simulink model "sim_PD"  (R2023a)
settings: Solver=VariableStepAuto  StartTime=0.0  StopTime=20  RelTol=1e-3
values from neighbouring files (symbols this model uses):
  Kd = ((4*Jeff)/A-Beff)/Km_R    [val.m]
  Kp = (4*Jeff)/(square(A)*Km_R)    [val.m]
  r = 1/200    (= 0.005)    [val.m]
libraries: lib_robotRP_new x2
settings Model: Creator=gbl3344a  LastModifiedBy=gbl3344a

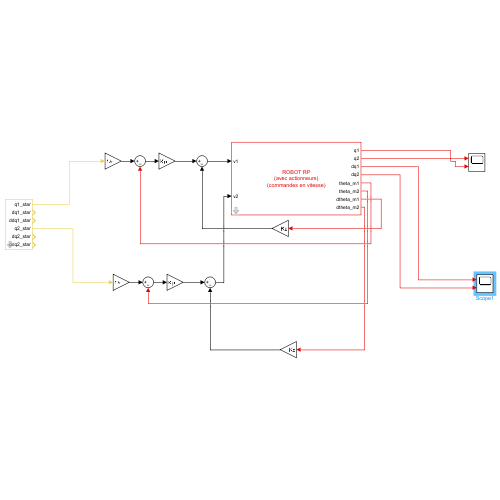
[thumbnail: Simulink's stored preview of the top-level diagram]
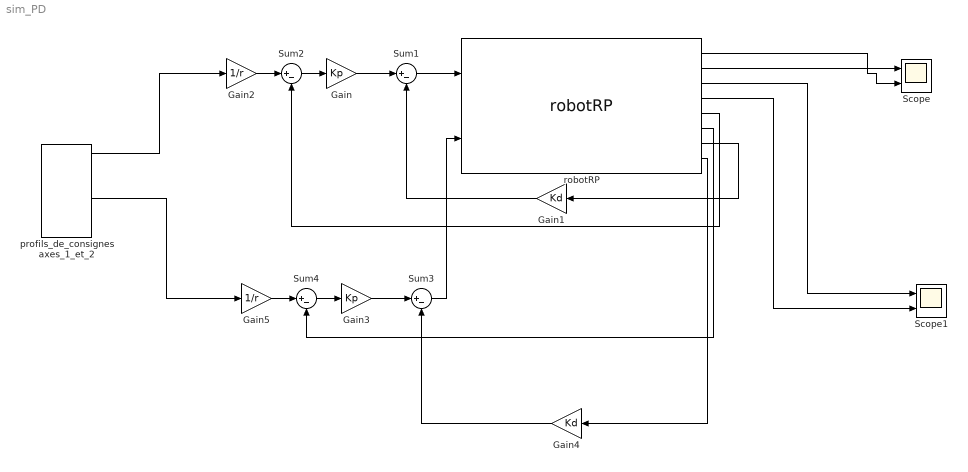
== system sim_PD ==
  Gain : Gain  Gain=Kp
  Gain1 : Gain  Gain=Kd
  Gain2 : Gain  Gain=1/r
  Gain3 : Gain  Gain=Kp
  Gain4 : Gain  Gain=Kd
  Gain5 : Gain  Gain=1/r
  Scope : Scope  NumInputPorts=2
  Scope1 : Scope  NumInputPorts=2
  Sum{1..4} (4 alike) : Sum  Inputs=|+-
  profils_de_consignes axes_1_et_2 : lib_robotRP_new/profils_de_consignes axes_1_et_2
  robotRP : lib_robotRP_new/robotRP  vecteur_theta_dtheta_initial=[0 ; 100 ; 0 ; 0]  m=15  gX=0  gY=-9.81  F1=0  F2=0  H1=0  H2=0  Km_sur_R=0.3  Jm=0.01  Beff=0.0125  r=1/30
  wires:
  Sum2/1 -> Gain/1
  Gain2/1 -> Sum2/1
  robotRP/1 -> Scope/2
  Gain1/1 -> Sum1/2
  Sum1/1 -> robotRP/1
  Gain/1 -> Sum1/1
  profils_de_consignes axes_1_et_2/1 -> Gain2/1
  Gain3/1 -> Sum3/1
  Gain4/1 -> Sum3/2
  Gain5/1 -> Sum4/1
  Sum4/1 -> Gain3/1
  Sum3/1 -> robotRP/2
  profils_de_consignes axes_1_et_2/4 -> Gain5/1
  robotRP/6 -> Sum4/2
  robotRP/8 -> Gain4/1
  robotRP/5 -> Sum2/2
  robotRP/7 -> Gain1/1
  robotRP/3 -> Scope1/1
  robotRP/4 -> Scope1/2
  robotRP/2 -> Scope/1
